simulink model "cruise_control"  (R2018b)
settings: Solver=VariableStepAuto  StartTime=0.0  StopTime=10.0  RelTol=1e-3
values from neighbouring files (symbols this model uses):
  const = vehicleConstants    [module2.m]
  Utrim = unperturb_controls    [TrimVehicle.m]    (also in module2.m = trimmed_control)
  Xtrim = unperturb_states    [TrimVehicle.m]    (also in module2.m = trimmed_state)
libraries: simulink x1
settings Model: Creator=rainli  LastModifiedBy=rainli

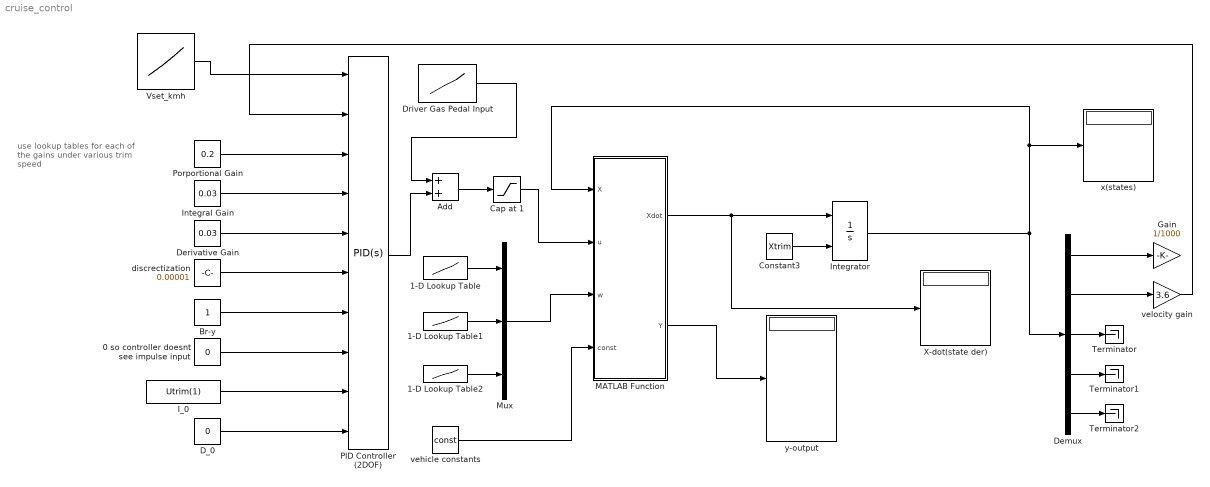
== system cruise_control ==
  note: use lookup tables for each of the gains under various trim speed
  "0 so controller doesnt see impulse input " : Constant  Value=0
  1-D Lookup Table : Lookup_n-D  NumberOfTableDimensions=1  BreakpointsForDimension1=[-5:5]  Table=tanh([-5:5])  InternalRulePriority=Speed  RndMeth=Simplest  InputSameDT=on
  1-D Lookup Table1 : Lookup_n-D  NumberOfTableDimensions=1  BreakpointsForDimension1=[-5:5]  Table=tanh([-5:5])  InternalRulePriority=Speed  RndMeth=Simplest  InputSameDT=on
  1-D Lookup Table2 : Lookup_n-D  NumberOfTableDimensions=1  BreakpointsForDimension1=[-5:5]  Table=tanh([-5:5])  InternalRulePriority=Speed  RndMeth=Simplest  InputSameDT=on
  Add : Sum
  Br-y : Constant
  Cap at 1 : Saturate  UpperLimit=1  LowerLimit=0
  Constant3 : Constant  Value=Xtrim
  D_0 : Constant  Value=0
  Demux : Demux  Outputs=5
  Derivative Gain : Constant  Value=0.03
  Driver Gas Pedal Input : Lookup_n-D  NumberOfTableDimensions=1  BreakpointsForDimension1=[-5:5]  Table=tanh([-5:5])  InternalRulePriority=Speed  RndMeth=Simplest  InputSameDT=on
  Gain : Gain  Gain=1/1000
  I_0 : Constant  Value=Utrim(1)
  Integral Gain : Constant  Value=0.03
  Integrator : Integrator  InitialConditionSource=external
  MATLAB Function : MATLAB Function  TreatAsAtomicUnit=on
  Mux : Mux  Inputs=3
  PID Controller (2DOF) : simulink/Continuous/PID Controller (2DOF)  Controller=PID  Form=Parallel  TimeDomain=Continuous-time  SampleTime=-1  IntegratorMethod=Forward Euler  FilterMethod=Forward Euler  ControllerParametersSource=external  P=1  I=1  D=0  UseFilter=on  N=100  b=1  c=1  TunerSelectOption=Transfer Function Based (PID Tuner App)  InitialConditionSource=external  InitialConditionForIntegrator=0  InitialConditionForFilter=0  DifferentiatorICPrevScaledInput=0  ExternalReset=none  TrackingMode=off  Kt=1  LimitOutput=on  UpperSaturationLimit=1  LowerSaturationLimit=0  LinearizeAsGain=on  AntiWindupMode=clamping  Kb=1  POutMin=[]  POutMax=[]  IOutMin=[]  IOutMax=[]  DOutMin=[]  DOutMax=[]  NOutMin=[]  NOutMax=[]  bOutMin=[]  bOutMax=[]  cOutMin=[]  cOutMax=[]  SumOutMin=[]  SumOutMax=[]  SaturationOutMin=[]  SaturationOutMax=[]  PParamMin=[]  PParamMax=[]  IParamMin=[]  IParamMax=[]  DParamMin=[]  DParamMax=[]  NParamMin=[]  NParamMax=[]  bParamMin=[]  bParamMax=[]  cParamMin=[]  cParamMax=[]  KbParamMin=[]  KbParamMax=[]  KtParamMin=[]  KtParamMax=[]  KbOutMin=[]  KbOutMax=[]  KtOutMin=[]  KtOutMax=[]  IntegratorOutMin=[]  IntegratorOutMax=[]  FilterOutMin=[]  FilterOutMax=[]  SumI1OutMin=[]  SumI1OutMax=[]  SumI2OutMin=[]  SumI2OutMax=[]  SumI3OutMin=[]  SumI3OutMax=[]  SumI4OutMin=[]  SumI4OutMax=[]  SumDOutMin=[]  SumDOutMax=[]  Sum1OutMin=[]  Sum1OutMax=[]  Sum2OutMin=[]  Sum2OutMax=[]  Sum3OutMin=[]  Sum3OutMax=[]  DifferentiatorOutMin=[]  DifferentiatorOutMax=[]  FilterDiffOutCoefMin=[]  FilterDiffOutCoefMax=[]  ReciprocalOutMin=[]  ReciprocalOutMax=[]  SumDenOutMin=[]  SumDenOutMax=[]  SumNumOutMin=[]  SumNumOutMax=[]  DivideOutMin=[]  DivideOutMax=[]  IntegratorContinuousStateAttributes=''  IntegratorStateMustResolveToSignalObject=off  IntegratorRTWStateStorageClass=Auto  FilterContinuousStateAttributes=''  FilterStateMustResolveToSignalObject=off  FilterRTWStateStorageClass=Auto  ParallelPVariant=ExternalParameters  IdealPVariant=Disabled  IVariant=ExternalParameters  DVariant=ExternalParameters  bVariant=ExternalParameters  cVariant=ExternalParameters  IntegratorVariant=Continuous  SatVariant=Enabled  AWVariant=ContClampingParallel  PCopyVariant=Disabled  TRVariant=Disabled  FdbkBlocksVariant=Forward  IdealPFdbkVariant=Disabled  SatFdbkVariant=Disabled  DerivativeFilterVariant=ContFilter  NVariant=ExternalParameters  NCopyVariant=Disabled  FilterICVariant=ExternalICs  IntegratorICVariant=ExternalICs  ExternalResetVariant=Disabled  TRSumVariant=Passthrough  SumFdbkVariant=Disabled  SumVariant=Sum_PID
  Porportional Gain : Constant  Value=0.2
  Terminator : Terminator
  Terminator1 : Terminator
  Terminator2 : Terminator
  Vset_kmh : Lookup_n-D  NumberOfTableDimensions=1  BreakpointsForDimension1=[-5:5]  Table=tanh([-5:5])  InternalRulePriority=Speed  RndMeth=Simplest  InputSameDT=on
  X-dot(state der) : Display
  discrectization : Constant  Value=0.00001
  vehicle constants : Constant  Value=const
  velocity gain : Gain  Gain=3.6
  x(states) : Display
  y-output : Display
  wires:
  MATLAB Function/1(Xdot) -> Integrator/1, X-dot(state der)/1
  MATLAB Function/2(Y) -> y-output/1
  Cap at 1/1 -> MATLAB Function/2(u)
  vehicle constants/1 -> MATLAB Function/4(const)
  Mux/1 -> MATLAB Function/3(w)
  Constant3/1 -> Integrator/2
  Integrator/1 -> x(states)/1, MATLAB Function/1(X), Demux/1
  Vset_kmh/1 -> PID Controller (2DOF)/1
  Demux/1 -> Gain/1
  Demux/2 -> velocity gain/1
  Demux/3 -> Terminator/1
  Demux/4 -> Terminator1/1
  Demux/5 -> Terminator2/1
  velocity gain/1 -> PID Controller (2DOF)/2
  Porportional Gain/1 -> PID Controller (2DOF)/3
  Integral Gain/1 -> PID Controller (2DOF)/4
  Derivative Gain/1 -> PID Controller (2DOF)/5
  Br-y/1 -> PID Controller (2DOF)/7
  "0 so controller doesnt see impulse input "/1 -> PID Controller (2DOF)/8
  discrectization/1 -> PID Controller (2DOF)/6
  I_0/1 -> PID Controller (2DOF)/9
  D_0/1 -> PID Controller (2DOF)/10
  PID Controller (2DOF)/1 -> Add/2
  Driver Gas Pedal Input/1 -> Add/1
  Add/1 -> Cap at 1/1
  1-D Lookup Table1/1 -> Mux/2
  1-D Lookup Table2/1 -> Mux/3
  1-D Lookup Table/1 -> Mux/1

== matlab function cruise_control/MATLAB Function ==
  data: X input; u input; Xdot output; w input; const input; Y output
function [Xdot,Y] = fcn(X,u,w,const)
[Xdot,Y] = VehicleDynamicsModel(X,u,w,const);
